simulink model "SimulinkModel"  (R2020b)
settings: Solver=VariableStepAuto  StartTime=0.0  StopTime=10.0  RelTol=1e-3
values from neighbouring files (symbols this model uses):
  B = 6*pi*r*mu    (= 0.000523565265277)    [ModelScript.m]    (also in Old_Multi_Bode.m = zeros(length(omega),1))
  Mp = rho_p * Vp    (= 5.13126800086e-09)    [ModelScript.m]
settings Model: Creator=wneum  LastModifiedBy=wneum

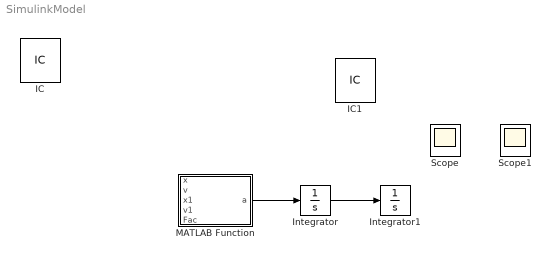
== system SimulinkModel ==
  IC : InitialCondition
  IC1 : InitialCondition
  Integrator : Integrator
  Integrator1 : Integrator
  MATLAB Function : MATLAB Function  TreatAsAtomicUnit=on
  Scope : Scope
  Scope1 : Scope
  wires:
  Integrator/1 -> Integrator1/1
  MATLAB Function/1(a) -> Integrator/1

== matlab function SimulinkModel/MATLAB Function ==
  data: x input; a output; v input; x1 input; v1 input; Fac input; Mp parameter; B parameter
function a = fcn(x,v,x1,v1,Fac, Mp, B)

a = 1/Mp * (Fac - B*v);
